simulink model "CH12_3B"  (R2021b)
settings: Solver=ode45  StartTime=0.0  StopTime=0.2  RelTol=1e-3
libraries: dsparch4 x3, simulink x1
settings Model: Creator=NA  LastModifiedBy=82102
settings SolverCC: AlgebraicLoopSolver=TrustRegion
settings DataIOCC: LimitDataPoints=on  SaveFormat=Array  SignalLoggingSaveFormat=ModelDataLogs  ReturnWorkspaceOutputs=off
settings OptimizationCC: BlockReduction=off  BooleanDataType=off  LifeSpan=inf
settings DebuggingCC: SaveWithParameterizedLinksMsg=none  UnderspecifiedInitializationDetection=Classic  MergeDetectMultiDrivingBlocksExec=none  SignalResolutionControl=TryResolveAllWithWarning  MultiTaskDSMMsg=warning  MultiTaskCondExecSysMsg=none  FcnCallInpInsideContextMsg=warning  SFUnexpectedBacktrackingDiag=warning  SFNoUnconditionalDefaultTransitionDiag=warning  SFExecutionAtInitializationDiag=none  SFMachineParentedDataDiag=warning  ArithmeticOperatorsInVariantConditions=warning
settings HardwareCC: ProdBitPerPointer=32  ProdBitPerSizeT=32  ProdBitPerPtrDiffT=32  ProdLargestAtomicFloat=None  ProdIntDivRoundTo=Undefined  ProdEndianess=Unspecified  ProdWordSize=32  ProdHWDeviceType=32-bit Generic  TargetUnknown=on
settings ModelReferenceCC: PropagateSignalLabelsOutOfModel=off
settings SFSimCC: SimUseLocalCustomCode=off  CustomCodeUndefinedFunction=UseInterfaceOnly
settings RTWCC: RTWUseLocalCustomCode=off
settings CodeAppCC: StateflowObjectComments=on
settings GRTTargetCC: TargetLangStandard=C89/C90 (ANSI)  CombineOutputUpdateFcns=off  GRTInterface=on
settings ConfigComp: CovMetricSettings=dw  CovSaveCumulativeToWorkspaceVar=on  CovSaveSingleToWorkspaceVar=on  CovExternalEMLEnable=off

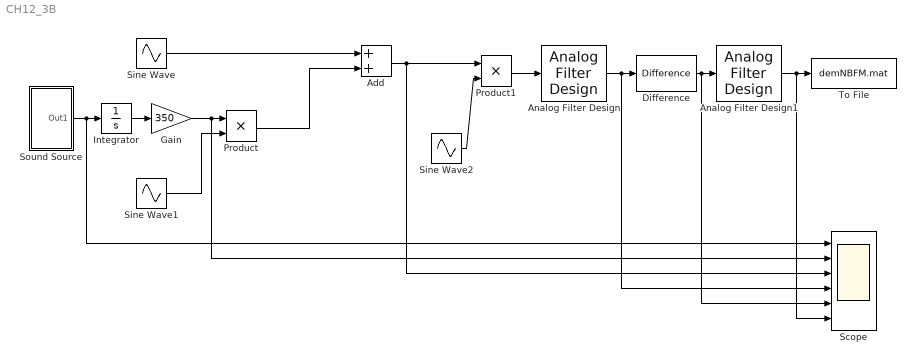
== system CH12_3B ==
  Add : Sum
  Analog Filter Design : dsparch4/Analog Filter Design  method=Butterworth  filttype=Lowpass  N=8  Wlo=2*pi*4e3  Whi=80  Rp=2  Rs=40
  Analog Filter Design1 : dsparch4/Analog Filter Design  method=Butterworth  filttype=Lowpass  N=8  Wlo=2*pi*4e3  Whi=80  Rp=2  Rs=40
  Difference : simulink/Discrete/Difference  ICPrevInput=0.0  OutMin=[]  OutMax=[]  OutDataType=fixdt(1, 16)  OutScaling=2^-10  DoSatur=off
  Gain : Gain  Gain=350
  Integrator : Integrator
  Product : Product
  Product1 : Product
  Scope : Scope  NumInputPorts=6
  Sine Wave : Sin  Frequency=2*pi*10e3  Phase=pi/2  SampleTime=0
  Sine Wave1 : Sin  Amplitude=-1  Frequency=2*pi*10e3  SampleTime=0
  Sine Wave2 : Sin  Amplitude=-1  Frequency=2*pi*10e3  SampleTime=0
  Sound Source : Subsystem
  To File : ToFile  Filename=demNBFM.mat  SampleTime=1/8192
  wires:
  Sound Source/1(Out1) -> Integrator/1, Scope/1
  Product1/1 -> Analog Filter Design/1
  Analog Filter Design/1 -> Scope/4, Difference/1
  Sine Wave2/1 -> Product1/2
  Integrator/1 -> Gain/1
  Gain/1 -> Scope/2, Product/1
  Sine Wave1/1 -> Product/2
  Sine Wave/1 -> Add/1
  Analog Filter Design1/1 -> Scope/6, To File/1
  Difference/1 -> Scope/5, Analog Filter Design1/1
  Add/1 -> Product1/1, Scope/3
  Product/1 -> Add/2

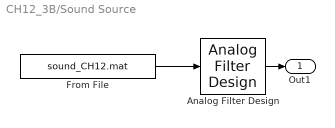
== system CH12_3B/Sound Source ==
  Analog Filter Design : dsparch4/Analog Filter Design  method=Butterworth  filttype=Lowpass  N=8  Wlo=4e3*2*pi  Whi=80  Rp=2  Rs=40
  From File : FromFile  FileName=sound_CH12.mat  SampleTime=0
  Out1 : Outport
  wires:
  From File/1 -> Analog Filter Design/1
  Analog Filter Design/1 -> Out1/1
